simulink model "IP_LQG_PCI6221_SwingUp"  (R2026a)
settings: Solver=VariableStepAuto
values from neighbouring files (symbols this model uses):
  ALPHA_MAX = 90  * pi/180    (= 1.57079632679)    [IP_MACRO.m]
  ALPHA_SWITCH = 30*pi/180    (= 0.523598775598)    [IP_MACRO.m]
  BETA_MAX = 15  * pi/180    (= 0.261799387799)    [IP_MACRO.m]
  g_acc = 9.81    [IP_MACRO.m]
  J2_nl = 0.004873    [IP_MACRO.m]
  K_aug = lqr(A_aug, B_aug, Qr_aug, Rr_aug)    [IP_MACRO.m]
  k_swingup = 10    [IP_MACRO.m]
  L = lqe(A, G, C, Qe, Re)    [IP_MACRO.m]
  lp = 0.1685    [IP_MACRO.m]
  mp = 0.127    [IP_MACRO.m]
  TIME_DELAY = 6    [IP_MACRO.m]
  Ts = 0.001    [IP_MACRO.m]
  V_MAX = 5    [IP_MACRO.m]
  V_MIN = -5    [IP_MACRO.m]
undefined symbols (not defined in the file or in its folder): A, B, C, National_Instruments, PCI
libraries: sldrtlib x3, simulink x2
settings Model: Creator=Tomas Teixeira  LastModifiedBy=Tomas Teixeira
settings DebuggingCC: MergeDetectMultiDrivingBlocksExec=error
settings ModelReferenceCC: PropagateSignalLabelsOutOfModel=on

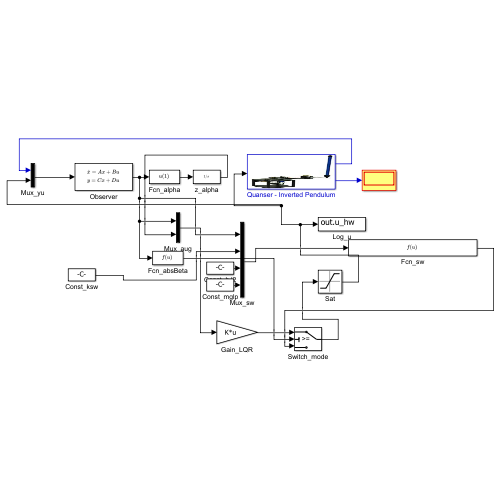
[thumbnail: Simulink's stored preview of the top-level diagram]
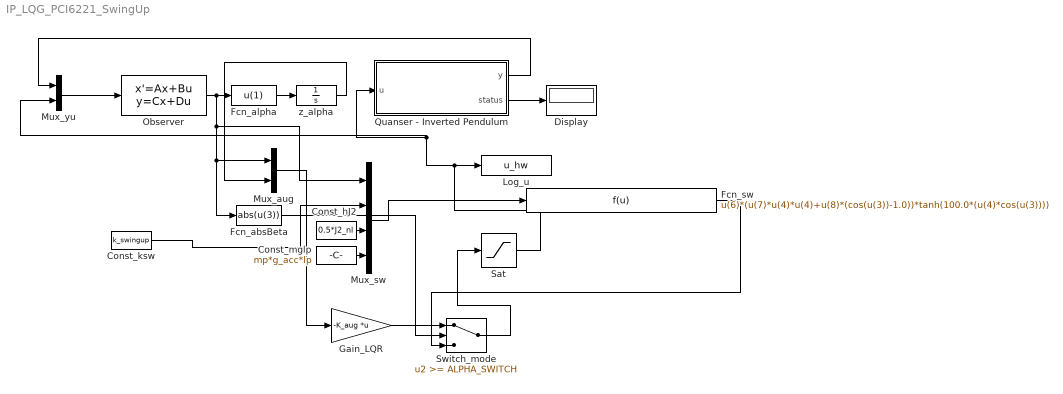
== system IP_LQG_PCI6221_SwingUp ==
  Const_hJ2 : Constant  Value=0.5*J2_nl
  Const_ksw : Constant  Value=k_swingup
  Const_mglp : Constant  Value=mp*g_acc*lp
  Display : Display
  Fcn_absBeta : Fcn  Expr=abs(u(3))
  Fcn_alpha : Fcn  Expr=u(1)
  Fcn_sw : Fcn  Expr=u(6)*(u(7)*u(4)*u(4)+u(8)*(cos(u(3))-1.0))*tanh(100.0*(u(4)*cos(u(3))))
  Gain_LQR : Gain  Gain=-K_aug  Multiplication=Matrix(K*u)
  Log_u : ToWorkspace  VariableName=u_hw  SampleTime=-1
  Mux_aug : Mux  Inputs=2
  Mux_sw : Mux
  Mux_yu : Mux  Inputs=2
  Observer : StateSpace  A=A-L*C  B=[L, B]  C=eye(5)  D=zeros(5,3)  InitialCondition=zeros(5,1)
  Quanser - Inverted Pendulum : Subsystem
      mask Display: image('IP_QUANSER.jpg');
  Sat : Saturate  UpperLimit=V_MAX  LowerLimit=V_MIN
  Switch_mode : Switch  Threshold=ALPHA_SWITCH  SaturateOnIntegerOverflow=off  InputSameDT=off
  z_alpha : Integrator
  wires:
  Quanser - Inverted Pendulum/1(y) -> Mux_yu/1
  Quanser - Inverted Pendulum/2(status) -> Display/1
  Mux_yu/1 -> Observer/1
  Observer/1 -> Mux_aug/1, Fcn_absBeta/1, Mux_sw/1, Fcn_alpha/1
  Fcn_alpha/1 -> z_alpha/1
  z_alpha/1 -> Mux_aug/2
  Mux_aug/1 -> Gain_LQR/1
  Gain_LQR/1 -> Switch_mode/1
  Const_ksw/1 -> Mux_sw/2
  Const_hJ2/1 -> Mux_sw/3
  Const_mglp/1 -> Mux_sw/4
  Mux_sw/1 -> Fcn_sw/1
  Fcn_sw/1 -> Switch_mode/3
  Fcn_absBeta/1 -> Switch_mode/2
  Switch_mode/1 -> Sat/1
  Sat/1 -> Quanser - Inverted Pendulum/1(u), Mux_yu/2, Log_u/1

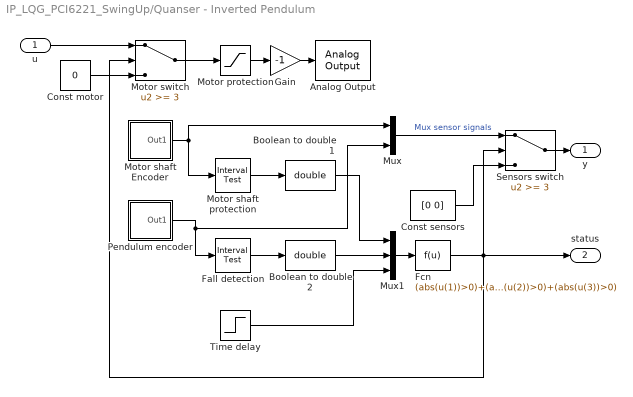
== system IP_LQG_PCI6221_SwingUp/Quanser - Inverted Pendulum ==
  u : Inport
  Analog Output : sldrtlib/Analog Output  SampleTime=Ts  MaxMissedTicks=10  ShowMissedTicks=off  YieldWhenWaiting=off  DrvName=National_Instruments/PCI-6221  DrvAddress=4294967295  DrvOptions=[0 0 0 2 2]  Channels=1  RangeMode=1  VoltRange=1  InitialValue=0  FinalValue=0
      settings: AttributesFormatString=National Instruments\nPCI-6221 [auto]
  Boolean to double 1 : DataTypeConversion  OutDataTypeStr=double  SaturateOnIntegerOverflow=off  RndMeth=Floor
  Boolean to double 2 : DataTypeConversion  OutDataTypeStr=double  SaturateOnIntegerOverflow=off  RndMeth=Floor
  Const motor : Constant  Value=0
  Const sensors : Constant  Value=[0 0]
  Fall detection : simulink/Logic and Bit Operations/Interval Test  IntervalClosedRight=on  uplimit=BETA_MAX  IntervalClosedLeft=on  lowlimit=-BETA_MAX  OutDataTypeStr=uint8
  Fcn : Fcn  Expr=(abs(u(1))>0)+(abs(u(2))>0)+(abs(u(3))>0)
  Gain : Gain  Gain=-1
  Motor protection : Saturate  UpperLimit=V_MAX  LowerLimit=V_MIN
  Motor shaft Encoder : Subsystem
  Motor shaft protection : simulink/Logic and Bit Operations/Interval Test  IntervalClosedRight=on  uplimit=ALPHA_MAX  IntervalClosedLeft=on  lowlimit=-ALPHA_MAX  OutDataTypeStr=uint8
  Motor switch : Switch  Threshold=3  SaturateOnIntegerOverflow=off  InputSameDT=off
  Mux : Mux  Inputs=2
  Mux1 : Mux  Inputs=3
  Pendulum encoder : Subsystem
  Sensors switch : Switch  Threshold=3  SaturateOnIntegerOverflow=off  InputSameDT=off
  Time delay : Step  Time=TIME_DELAY  SampleTime=0
  y : Outport
  status : Outport  Port=2
  wires:
  Motor protection/1 -> Gain/1
  Gain/1 -> Analog Output/1
  Sensors switch/1 -> y/1
  Mux/1 -> Sensors switch/1  "Mux sensor signals"
  Const sensors/1 -> Sensors switch/3
  Boolean to double 1/1 -> Mux1/1
  Motor shaft protection/1 -> Boolean to double 1/1
  Boolean to double 2/1 -> Mux1/2
  Fall detection/1 -> Boolean to double 2/1
  Time delay/1 -> Mux1/3
  Fcn/1 -> Motor switch/2, status/1, Sensors switch/2
  Mux1/1 -> Fcn/1
  Pendulum encoder/1(Out1) -> Mux/2, Fall detection/1
  Motor shaft Encoder/1(Out1) -> Motor shaft protection/1, Mux/1
  Const motor/1 -> Motor switch/3
  Motor switch/1 -> Motor protection/1
  u/1 -> Motor switch/1

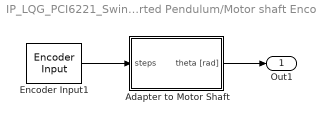
== system IP_LQG_PCI6221_SwingUp/Quanser - Inverted Pendulum/Motor shaft Encoder ==
  Adapter to Motor Shaft : Subsystem
  Encoder Input1 : sldrtlib/Encoder Input  SampleTime=Ts  MaxMissedTicks=inf  ShowMissedTicks=off  YieldWhenWaiting=off  DrvName=National_Instruments/PCI-6221  DrvAddress=4294967295  DrvOptions=[0 0 0 2 2]  Channels=1  QuadMode=3  IndexPulse=2  InputFilter=Inf  DataType=1
      settings: AttributesFormatString=National Instruments\nPCI-6221 [auto]
  Out1 : Outport
  wires:
  Adapter to Motor Shaft/1(theta [rad]) -> Out1/1
  Encoder Input1/1 -> Adapter to Motor Shaft/1(steps)

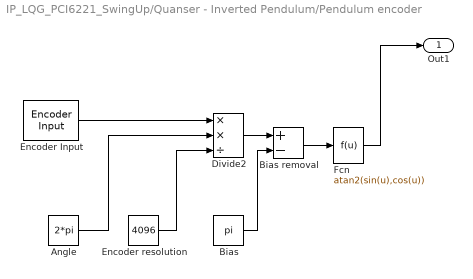
== system IP_LQG_PCI6221_SwingUp/Quanser - Inverted Pendulum/Pendulum encoder ==
  Angle : Constant  Value=2*pi
  Bias : Constant  Value=pi
  Bias removal : Sum  Inputs=+-
  Divide2 : Product  Inputs=**/
  Encoder resolution : Constant  Value=4096
  Encoder Input : sldrtlib/Encoder Input  SampleTime=Ts  MaxMissedTicks=inf  ShowMissedTicks=off  YieldWhenWaiting=off  DrvName=National_Instruments/PCI-6221  DrvAddress=4294967295  DrvOptions=[0 0 0 2 2]  Channels=2  QuadMode=3  IndexPulse=2  InputFilter=Inf  DataType=1
      settings: AttributesFormatString=National Instruments\nPCI-6221 [auto]
  Fcn : Fcn  Expr=atan2(sin(u),cos(u))
  Out1 : Outport
  wires:
  Angle/1 -> Divide2/2
  Bias removal/1 -> Fcn/1
  Encoder Input/1 -> Divide2/1
  Fcn/1 -> Out1/1
  Divide2/1 -> Bias removal/1
  Encoder resolution/1 -> Divide2/3
  Bias/1 -> Bias removal/2

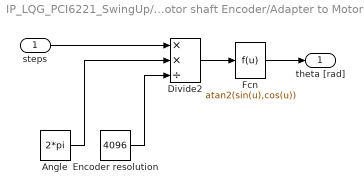
== system IP_LQG_PCI6221_SwingUp/Quanser - Inverted Pendulum/Motor shaft Encoder/Adapter to Motor Shaft ==
  steps : Inport
  Angle : Constant  Value=2*pi
  Divide2 : Product  Inputs=**/
  Encoder resolution : Constant  Value=4096
  Fcn : Fcn  Expr=atan2(sin(u),cos(u))
  theta [rad] : Outport
  wires:
  Fcn/1 -> theta [rad]/1
  Divide2/1 -> Fcn/1
  steps/1 -> Divide2/1
  Encoder resolution/1 -> Divide2/3
  Angle/1 -> Divide2/2
